simulink model "pressurizer"  (R2016a)
settings: Solver=VariableStepAuto  StartTime=0.0  StopTime=10.0  RelTol=1e-3
values from neighbouring files (symbols this model uses):
  c_p_PC = 5415    [unit_1.m]
  c_p_PR = 6873.1    [unit_1.m]
  c_phi_1 = 2.98    [unit_1.m]
  c_phi_2 = -0.008448    [unit_1.m]
  m_in = 1.4222    [unit_1.m]
  m_out = 2.9722    [unit_1.m]
  T_PC = 293.03    [unit_1.m]
  T_PC_HL = 293.08    [unit_1.m]
  V0_PC = 242    [unit_1.m]
  W_heat_PR = 1    [unit_1.m]
  W_loss_PR = 1.6823 * 10^5    (= 168230)    [unit_1.m]
undefined symbols (not defined in the file or in its folder): X_mPR_gtz, X_mPR_ltz
settings Model: Creator=Michal Chruscinski  LastModifiedBy=Michal Chruscinski
settings GRTTargetCC: GeneratePreprocessorConditionals=Use local settings

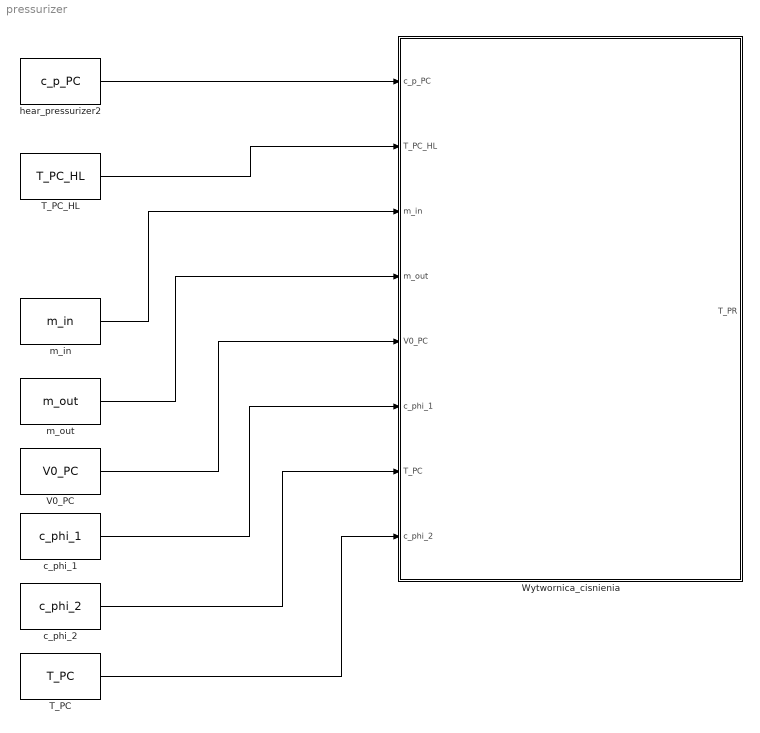
== system pressurizer ==
  T_PC : Constant  Value=T_PC
  T_PC_HL : Constant  Value=T_PC_HL
  V0_PC : Constant  Value=V0_PC
  Wytwornica_cisnienia : Subsystem
  c_phi_1 : Constant  Value=c_phi_1
  c_phi_2 : Constant  Value=c_phi_2
  hear_pressurizer2 : Constant  Value=c_p_PC
  m_in : Constant  Value=m_in
  m_out : Constant  Value=m_out
  wires:
  c_phi_2/1 -> Wytwornica_cisnienia/7(T_PC)
  T_PC/1 -> Wytwornica_cisnienia/8(c_phi_2)
  hear_pressurizer2/1 -> Wytwornica_cisnienia/1(c_p_PC)
  T_PC_HL/1 -> Wytwornica_cisnienia/2(T_PC_HL)
  m_in/1 -> Wytwornica_cisnienia/3(m_in)
  m_out/1 -> Wytwornica_cisnienia/4(m_out)
  V0_PC/1 -> Wytwornica_cisnienia/5(V0_PC)
  c_phi_1/1 -> Wytwornica_cisnienia/6(c_phi_1)

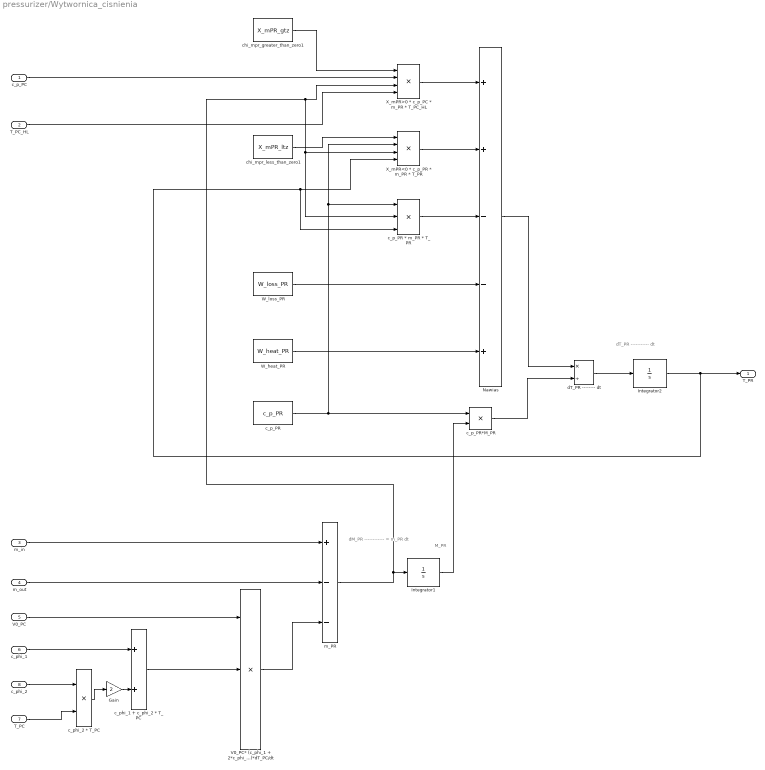
== system pressurizer/Wytwornica_cisnienia ==
  note: dT_PR
      | -----------
      | dt
  note: dM_PR
      | ------------ = m_PR
      |     dt
  note: M_PR
  c_p_PC : Inport
  T_PC_HL : Inport  Port=2
  m_in : Inport  Port=3
  m_out : Inport  Port=4
  V0_PC : Inport  Port=5
  c_phi_1 : Inport  Port=6
  T_PC : Inport  Port=7
  c_phi_2 : Inport  Port=8
  Gain : Gain  Gain=2
  Integrator1 : Integrator
  Integrator2 : Integrator
  Nawias : Sum  Inputs=++--+
  V0_PC* (c_phi_1 + 2*c_phi_2*T_PC)*dT_PC/dt : Product  Inputs=3
  W_heat_PR : Constant  Value=W_heat_PR
  W_loss_PR : Constant  Value=W_loss_PR
  X_mPR<0 * c_p_PR * m_PR * T_PR : Product  Inputs=4
  X_mPR>0 * c_p_PC * m_PR * T_PC_HL : Product  Inputs=4
  c_p_PR : Constant  Value=c_p_PR
  c_p_PR * m_PR * T_PR : Product  Inputs=3
  c_p_PR*M_PR : Product
  "c_phi_1 + c_phi_2 * T_PC " : Sum
  c_phi_2 * T_PC : Product
  chi_mpr_greater_than_zero1 : Constant  Value=X_mPR_gtz
  chi_mpr_less_than_zero1 : Constant  Value=X_mPR_ltz
  dT_PR -------- dt : Product  Inputs=*/
  m_PR : Sum  Inputs=+--
  T_PR : Outport
  wires:
  c_p_PR*M_PR/1 -> dT_PR -------- dt/2
  Nawias/1 -> dT_PR -------- dt/1
  Integrator1/1 -> c_p_PR*M_PR/2
  c_p_PR/1 -> X_mPR<0 * c_p_PR * m_PR * T_PR/2, c_p_PR * m_PR * T_PR/1, c_p_PR*M_PR/1
  chi_mpr_greater_than_zero1/1 -> X_mPR>0 * c_p_PC * m_PR * T_PC_HL/1
  X_mPR>0 * c_p_PC * m_PR * T_PC_HL/1 -> Nawias/1
  c_p_PC/1 -> X_mPR>0 * c_p_PC * m_PR * T_PC_HL/2
  m_PR/1 -> X_mPR>0 * c_p_PC * m_PR * T_PC_HL/3, c_p_PR * m_PR * T_PR/2, X_mPR<0 * c_p_PR * m_PR * T_PR/3, Integrator1/1
  T_PC_HL/1 -> X_mPR>0 * c_p_PC * m_PR * T_PC_HL/4
  X_mPR<0 * c_p_PR * m_PR * T_PR/1 -> Nawias/2
  chi_mpr_less_than_zero1/1 -> X_mPR<0 * c_p_PR * m_PR * T_PR/1
  Integrator2/1 -> X_mPR<0 * c_p_PR * m_PR * T_PR/4, c_p_PR * m_PR * T_PR/3, T_PR/1
  c_p_PR * m_PR * T_PR/1 -> Nawias/3
  W_heat_PR/1 -> Nawias/5
  W_loss_PR/1 -> Nawias/4
  m_in/1 -> m_PR/1
  m_out/1 -> m_PR/2
  V0_PC* (c_phi_1 + 2*c_phi_2*T_PC)*dT_PC/dt/1 -> m_PR/3
  V0_PC/1 -> V0_PC* (c_phi_1 + 2*c_phi_2*T_PC)*dT_PC/dt/1
  "c_phi_1 + c_phi_2 * T_PC "/1 -> V0_PC* (c_phi_1 + 2*c_phi_2*T_PC)*dT_PC/dt/2
  c_phi_1/1 -> "c_phi_1 + c_phi_2 * T_PC "/1
  c_phi_2 * T_PC/1 -> Gain/1
  Gain/1 -> "c_phi_1 + c_phi_2 * T_PC "/2
  c_phi_2/1 -> c_phi_2 * T_PC/1
  T_PC/1 -> c_phi_2 * T_PC/2
  dT_PR -------- dt/1 -> Integrator2/1
